simulink model "Lab04S"  (R2023b)
settings: Solver=VariableStepAuto  StartTime=0.0  StopTime=1  RelTol=1e-3
values from neighbouring files (symbols this model uses):
  A = [0 -1 5; 0 0 3; 0 0 -2]    [Lab01.m]    (also in Lab03.m = double(subs(A,x,x_eq)); Lab04.m = double(subs(A,[x u],[x_eq u_eq])); Lab05.m = [0 1; -3 -4])
  alpha = inv(-C*((A-B*K)\B))    [Lab04.m]    (also in Lab05.m; Prob1.m = 0.05; Prob2.m = 0.05; Prob3.m = 0.05)
  B = [1 1 1]'    [Lab01.m]    (also in Lab03.m = double(subs(B,u,u_eq)); Lab04.m = double(subs(B,[x u],[x_eq u_eq])); Lab05.m = [0 ; 1])
  C = [0 0 5]    [Lab01.m]    (also in Lab03.m = double(subs(C,x,x_eq)); Lab04.m = double(subs(C,x,x_eq)); Lab05.m = [2 1])
  D = double(subs(D,u,u_eq))    [Lab03.m]    (also in Lab04.m; Lab05.m = 0)
  G = 9.81    [Lab04.m]
  K = place(A,B,lambda_k)    [Lab04.m]    (also in Lab05.m)
  Km = 1.52*10^-4    (= 0.000152)    [Lab04.m]
  Kt = 708.27    [Lab04.m]
  L = place(A',C',lambda_o)'    [Lab04.m]    (also in Lab05.m; Prob1.m = -Kc*Gp*Ga; Prob2.m = -Kc*Gp*Ga; Prob3.m = -Kc*Gp*Ga)
  m = 0.02    [Lab04.m]
  u_eq = [r_eq gamma_eq]    [Lab03.m]    (also in Lab04.m = 0.8)
  x_eq = double([ G_eq I_eq beta_eq ])    [Lab03.m]    (also in Lab04.m = x_eq(2,:))
settings Model: Creator=matteo  LastModifiedBy=matteo

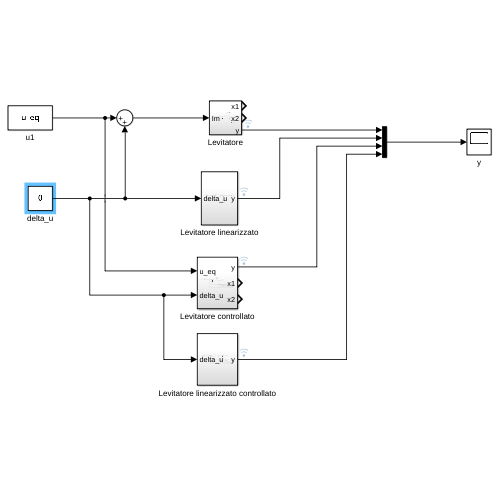
[thumbnail: Simulink's stored preview of the top-level diagram]
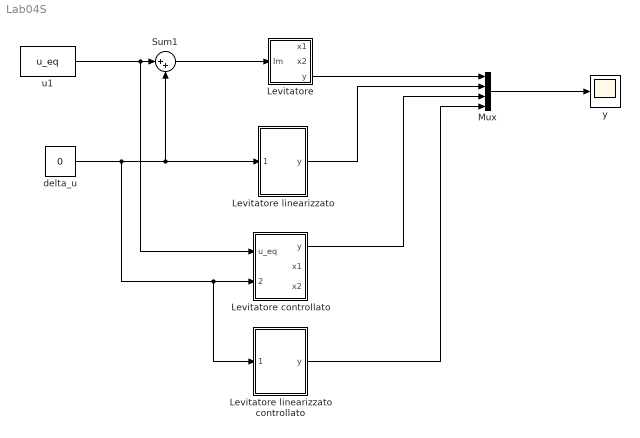
== system Lab04S ==
  Levitatore : Subsystem
  Levitatore controllato : Subsystem
  Levitatore linearizzato : Subsystem
  Levitatore linearizzato controllato : Subsystem
  Mux : Mux
  Sum1 : Sum  Inputs=|++
  delta_u : Constant  Value=0
  u1 : Constant  Value=u_eq
  y : Scope
  wires:
  u1/1 -> Levitatore controllato/1(u_eq), Sum1/1
  Sum1/1 -> Levitatore/1(Im)
  delta_u/1 -> Levitatore controllato/2(delta_u), Levitatore linearizzato controllato/1(delta_u), Levitatore linearizzato/1(delta_u), Sum1/2
  Levitatore/3(y) -> Mux/1
  Mux/1 -> y/1
  Levitatore controllato/1(y) -> Mux/3
  Levitatore linearizzato controllato/1(y) -> Mux/4
  Levitatore linearizzato/1(y) -> Mux/2

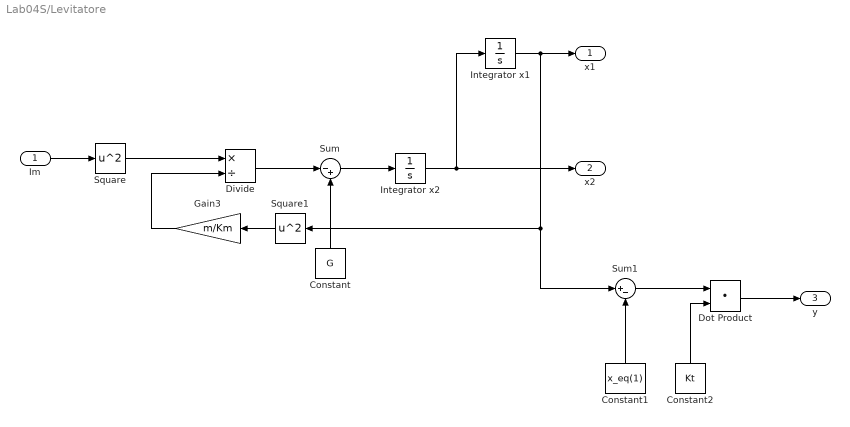
== system Lab04S/Levitatore ==
  Im : Inport
  Constant : Constant  Value=G
  Constant1 : Constant  Value=x_eq(1)
  Constant2 : Constant  Value=Kt
  Divide : Product  Inputs=*/
  Dot Product : DotProduct  OutDataTypeStr=Inherit: Inherit via internal rule
  Gain3 : Gain  Gain=m/Km
  Integrator x1 : Integrator  InitialCondition=x_eq(1)
  Integrator x2 : Integrator  InitialCondition=x_eq(2)
  Square : Math  Operator=square
  Square1 : Math  Operator=square
  Sum : Sum  Inputs=|-+
  Sum1 : Sum  Inputs=|+-
  x1 : Outport
  x2 : Outport  Port=2
  y : Outport  Port=3
  wires:
  Im/1 -> Square/1
  Constant/1 -> Sum/2
  Sum/1 -> Integrator x2/1
  Integrator x2/1 -> Integrator x1/1, x2/1
  Constant1/1 -> Sum1/2
  Sum1/1 -> Dot Product/1
  Constant2/1 -> Dot Product/2
  Dot Product/1 -> y/1
  Integrator x1/1 -> Sum1/1, Square1/1, x1/1
  Square/1 -> Divide/1
  Square1/1 -> Gain3/1
  Gain3/1 -> Divide/2
  Divide/1 -> Sum/1

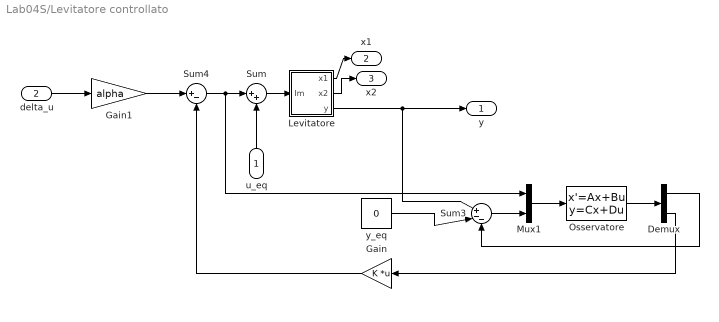
== system Lab04S/Levitatore controllato ==
  u_eq : Inport
  delta_u : Inport  Port=2
  Demux : Demux  Outputs=2
  Gain : Gain  Gain=K  Multiplication=Matrix(K*u)
  Gain1 : Gain  Gain=alpha
  Levitatore : Subsystem
  Mux1 : Mux  Inputs=2
  Osservatore : StateSpace  A=A  B=[B L]  C=[C; eye(2)]  D=zeros(3,2)  InitialCondition=0
  Sum : Sum  Inputs=|++
  Sum3 : Sum  Inputs=|+--
  Sum4 : Sum  Inputs=|+-
  y_eq : Constant  Value=0
  y : Outport
  x1 : Outport  Port=2
  x2 : Outport  Port=3
  wires:
  Sum/1 -> Levitatore/1(Im)
  Demux/2 -> Gain/1
  Levitatore/1(x1) -> x1/1
  delta_u/1 -> Gain1/1
  Sum3/1 -> Mux1/2
  Gain/1 -> Sum4/2
  Levitatore/3(y) -> Sum3/1, y/1
  Osservatore/1 -> Demux/1
  Sum4/1 -> Mux1/1, Sum/1
  Mux1/1 -> Osservatore/1
  u_eq/1 -> Sum/2
  Levitatore/2(x2) -> x2/1
  Gain1/1 -> Sum4/1
  Demux/1 -> Sum3/3
  y_eq/1 -> Sum3/2

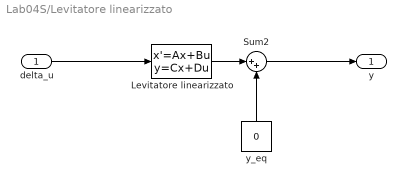
== system Lab04S/Levitatore linearizzato ==
  delta_u : Inport
  Levitatore linearizzato : StateSpace  A=A  B=B  C=C  D=D  InitialCondition=x_eq
  Sum2 : Sum  Inputs=|++
  y_eq : Constant  Value=0
  y : Outport
  wires:
  Levitatore linearizzato/1 -> Sum2/1
  Sum2/1 -> y/1
  y_eq/1 -> Sum2/2
  delta_u/1 -> Levitatore linearizzato/1

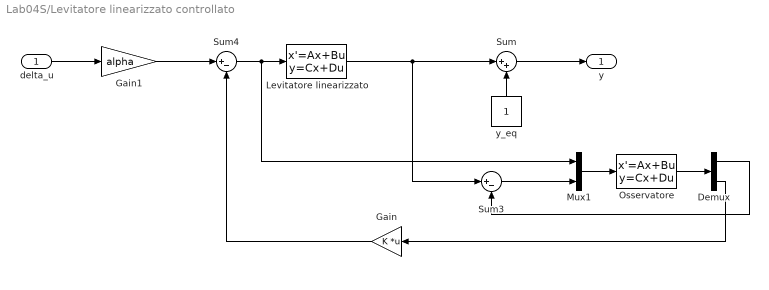
== system Lab04S/Levitatore linearizzato controllato ==
  delta_u : Inport
  Demux : Demux  Outputs=2
  Gain : Gain  Gain=K  Multiplication=Matrix(K*u)
  Gain1 : Gain  Gain=alpha
  Levitatore linearizzato : StateSpace  A=A  B=B  C=C  D=D  InitialCondition=x_eq
  Mux1 : Mux  Inputs=2
  Osservatore : StateSpace  A=A  B=[B L]  C=[C; eye(2)]  D=zeros(3,2)  InitialCondition=0
  Sum : Sum  Inputs=|++
  Sum3 : Sum  Inputs=|+-
  Sum4 : Sum  Inputs=|+-
  y_eq : Constant
  y : Outport
  wires:
  Demux/2 -> Gain/1
  delta_u/1 -> Gain1/1
  Sum3/1 -> Mux1/2
  Gain/1 -> Sum4/2
  Levitatore linearizzato/1 -> Sum/1, Sum3/1
  Osservatore/1 -> Demux/1
  Sum4/1 -> Levitatore linearizzato/1, Mux1/1
  Mux1/1 -> Osservatore/1
  Gain1/1 -> Sum4/1
  Demux/1 -> Sum3/2
  Sum/1 -> y/1
  y_eq/1 -> Sum/2

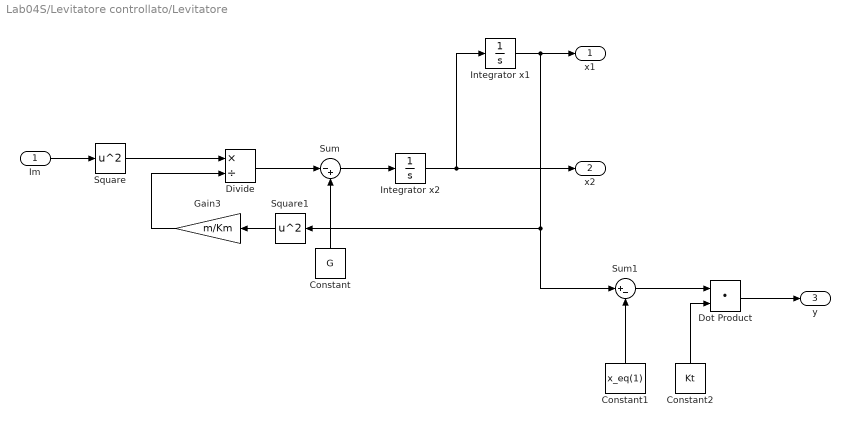
== system Lab04S/Levitatore controllato/Levitatore ==
  Im : Inport
  Constant : Constant  Value=G
  Constant1 : Constant  Value=x_eq(1)
  Constant2 : Constant  Value=Kt
  Divide : Product  Inputs=*/
  Dot Product : DotProduct  OutDataTypeStr=Inherit: Inherit via internal rule
  Gain3 : Gain  Gain=m/Km
  Integrator x1 : Integrator  InitialCondition=x_eq(1)
  Integrator x2 : Integrator  InitialCondition=x_eq(2)
  Square : Math  Operator=square
  Square1 : Math  Operator=square
  Sum : Sum  Inputs=|-+
  Sum1 : Sum  Inputs=|+-
  x1 : Outport
  x2 : Outport  Port=2
  y : Outport  Port=3
  wires:
  Im/1 -> Square/1
  Constant/1 -> Sum/2
  Sum/1 -> Integrator x2/1
  Integrator x2/1 -> Integrator x1/1, x2/1
  Constant1/1 -> Sum1/2
  Sum1/1 -> Dot Product/1
  Constant2/1 -> Dot Product/2
  Dot Product/1 -> y/1
  Integrator x1/1 -> Sum1/1, Square1/1, x1/1
  Square/1 -> Divide/1
  Square1/1 -> Gain3/1
  Gain3/1 -> Divide/2
  Divide/1 -> Sum/1
